simulink model "func7"  (R2020a)
settings: Solver=VariableStepAuto  StartTime=0.0  StopTime=10.0  RelTol=1e-3  EnableMultiTasking=on
undefined symbols (not defined in the file or in its folder): S, vsva2197, xcvc1902
libraries: ModelComposer x3, templatized_input_7_lib x2
settings Model: Creator=viswanad  LastModifiedBy=viswanad
settings DataIOCC: ReturnWorkspaceOutputs=off
settings OptimizationCC: LifeSpan=inf
settings DebuggingCC: SFUnexpectedBacktrackingDiag=warning  SFNoUnconditionalDefaultTransitionDiag=warning  ArithmeticOperatorsInVariantConditions=warning
settings SFSimCC: SimUseLocalCustomCode=off  CustomCodeUndefinedFunction=UseInterfaceOnly
settings RTWCC: RTWUseLocalCustomCode=off
settings CodeAppCC: StateflowObjectComments=on
settings GRTTargetCC: TargetLangStandard=C89/C90 (ANSI)
settings ConfigComp: CovMetricSettings=dw  CovHtmlReporting=on  CovSaveCumulativeToWorkspaceVar=on  CovSaveSingleToWorkspaceVar=on  CovExternalEMLEnable=off

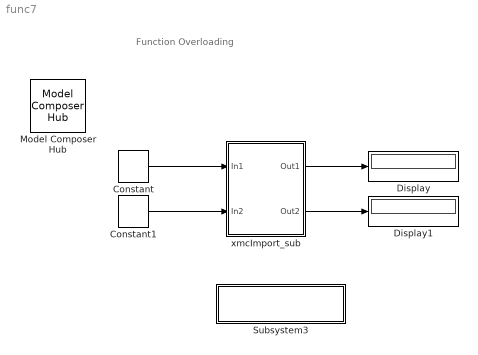
== system func7 ==
  note: Function Overloading
  Constant : ModelComposer/Constant  Value=-12  VectorParams1D=off  SampleTime=1  OutDataType=int16  TypeExp=''  Signedness=Signed  WordLength=16  FractionalLength=0  RoundingMode=Truncation to minus infinity  OverflowMode=Wrap around
  Constant1 : ModelComposer/Constant  Value=-2.4  VectorParams1D=off  SampleTime=1  OutDataType=fixed  TypeExp=''  Signedness=Signed  WordLength=16  FractionalLength=6  RoundingMode=Truncation to minus infinity  OverflowMode=Wrap around
  Display : Display
  Display1 : Display
  Model Composer Hub : ModelComposer/Model Composer Hub  CodeGeneration=off  SubsystemName=xmcImport_sub  TargetDirectory=./code  ExportType=IP Catalog  IpVendor=xilinx.com  IpLibrary=hls  IpVersion=1.0  IpHWLanguage=Verilog  AieCompilerOptions={}  CreateTestbench=off  TestbenchStackSize=10  RunAieSim=off  AieSimTimeout=50000  RunAieSimProfiling=off  LaunchVitisAnalyzer=off  PlotOutput=off  RunX86Sim=off  X86SimTimeout=10  GenHwImage=off  PlatformType=Not Specified  ProjDevice=xcvc1902-vsva2197-2MP-e-S  ProjDevicePart=xcvc1902-vsva2197-2MP-e-S  SamplePeriod=-1  ClockFrequency=200  DataPathParallelism=1
  Subsystem3 : Subsystem
      settings: OpenFcn=xmcOpenFileEx
      mask Display: disp(sprintf('Double Click to open\nthe main header file'))
  xmcImport_sub : Subsystem
  wires:
  Constant/1 -> xmcImport_sub/1(In1)
  Constant1/1 -> xmcImport_sub/2(In2)
  xmcImport_sub/1(Out1) -> Display/1
  xmcImport_sub/2(Out2) -> Display1/1

== system func7/Subsystem3 ==

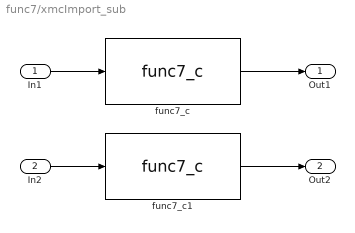
== system func7/xmcImport_sub ==
  In1 : Inport
  In2 : Inport  Port=2
  func7_c : templatized_input_7_lib/func7_c  LibraryFunction=func7_c  IncludeFiles={'func7_c.h'}  SourceFiles={}  IncludeDirectories={}  TemplateParams={{' '}, {' '}}  FunctionParamTypes={{xmcDataType('int16_t'); xmcDataType('int16_t')}, {xmcDataType('ap_fixed<16, 10>'); xmcDataType('ap_fixed<16, 10>')}}  FunctionParamPassbys={{0.000000000000000000e+00; 0.000000000000000000e+00}, {0.000000000000000000e+00; 0.000000000000000000e+00}}  FunctionParamDimensions={{'1'; '1'}, {'1'; '1'}}  FunctionParamNames={{'return'; 'var'}, {'return'; 'var'}}  FunctionParamDir={{2.000000000000000000e+00; 1.000000000000000000e+00}, {2.000000000000000000e+00; 1.000000000000000000e+00}}  FunctionParamSupportsStreaming={{false; false}, {false; false}}  BufferDepth={{'0'}, {'0'}}  FunctionParamValues={{'0'; '0'}, {'0'; '0'}}  ThroughputFactors={{''}, {''}}
  func7_c1 : templatized_input_7_lib/func7_c  LibraryFunction=func7_c  IncludeFiles={'func7_c.h'}  SourceFiles={}  IncludeDirectories={}  TemplateParams={{' '}, {' '}}  FunctionParamTypes={{xmcDataType('int16_t'); xmcDataType('int16_t')}, {xmcDataType('ap_fixed<16, 10>'); xmcDataType('ap_fixed<16, 10>')}}  FunctionParamPassbys={{0.000000000000000000e+00; 0.000000000000000000e+00}, {0.000000000000000000e+00; 0.000000000000000000e+00}}  FunctionParamDimensions={{'1'; '1'}, {'1'; '1'}}  FunctionParamNames={{'return'; 'var'}, {'return'; 'var'}}  FunctionParamDir={{2.000000000000000000e+00; 1.000000000000000000e+00}, {2.000000000000000000e+00; 1.000000000000000000e+00}}  FunctionParamSupportsStreaming={{false; false}, {false; false}}  BufferDepth={{'0'}, {'0'}}  FunctionParamValues={{'0'; '0'}, {'0'; '0'}}  ThroughputFactors={{''}, {''}}
  Out1 : Outport
  Out2 : Outport  Port=2
  wires:
  In2/1 -> func7_c1/1
  func7_c/1 -> Out1/1
  In1/1 -> func7_c/1
  func7_c1/1 -> Out2/1
